simulink model "Nolineal_Primer_Orden"  (R2017a)
settings: Solver=VariableStepAuto  StartTime=0.0  StopTime=20  RelTol=1e-3
settings Model: Creator=doctorado  LastModifiedBy=doctorado

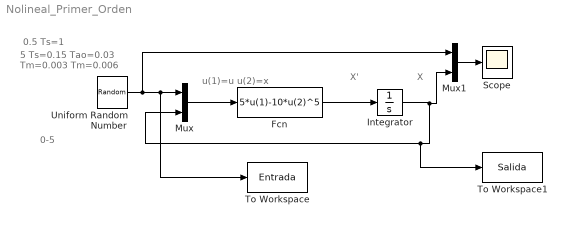
== system Nolineal_Primer_Orden ==
  note: 5 Ts=0.15
      | Tao=0.03
      | Tm=0.003
      | Tm=0.006
  note: 0.5 Ts=1
  note: 0-5
  note: u(1)=u
      | u(2)=x
  note: X
  note: X'
  Fcn : Fcn  Expr=5*u(1)-10*u(2)^5
  Integrator : Integrator
  Mux : Mux  Inputs=2
  Mux1 : Mux  Inputs=2
  Scope : Scope
  To Workspace : ToWorkspace  VariableName=Entrada  SampleTime=0.006
  To Workspace1 : ToWorkspace  VariableName=Salida  SampleTime=0.006
  Uniform Random Number : UniformRandomNumber  Minimum=0  Maximum=5  SampleTime=1
  wires:
  Fcn/1 -> Integrator/1
  Mux/1 -> Fcn/1
  Integrator/1 -> Mux1/2, To Workspace1/1, Mux/2
  Uniform Random Number/1 -> Mux1/1, To Workspace/1, Mux/1
  Mux1/1 -> Scope/1
